simulink model "Roll_OpenLoop"  (R2016b)
settings: Solver=ode3  StartTime=0.0  StopTime=10  FixedStep=.02  RelTol=1e-3  EnableMultiTasking=on
InitFcn:
  | close all
  | clear
  | clc
  | Parameter_Modeling
  | ST=0.02;
  | angle_scale=.0109863;  % 1/91.0222
  | time_scale=.01;
undefined symbols (not defined in the file or in its folder): rad, s
libraries: arduinolib x6, aerolibconvert2 x4, simulink x1
settings Model: SimulationMode=external  ExtModeTrigDuration=2  Creator=Alireza  LastModifiedBy=Ali
settings DataIOCC: LimitDataPoints=on  SaveFormat=Array
settings OptimizationCC: ExpressionDepthLimit=2147483647  MaxStackSize=64
settings DebuggingCC: UnderspecifiedInitializationDetection=Classic  MergeDetectMultiDrivingBlocksExec=none  ParameterTunabilityLossMsg=error  StateNameClashWarn=warning  SFUnexpectedBacktrackingDiag=warning  SFNoUnconditionalDefaultTransitionDiag=warning  SFExecutionAtInitializationDiag=none
settings HardwareCC: ProdBitPerInt=16  ProdBitPerPointer=16  ProdBitPerSizeT=16  ProdBitPerPtrDiffT=16  ProdLargestAtomicFloat=None  ProdWordSize=8  ProdHWDeviceType=Atmel->AVR
settings ModelReferenceCC: PropagateSignalLabelsOutOfModel=off
settings RTWCC: SystemTargetFile=ert.tlc  HardwareBoard=Arduino Mega 2560  TLCOptions=-aInlineSetEventsForThisBaseRateFcn=TLC_FALSE -aRateBasedStepFcn=1 -aSuppressMultiTaskScheduler=TLC_FALSE  TemplateMakefile=ert_default_tmf  Description=Embedded Coder  GenerateReport=on  RTWVerbose=off  Toolchain=Arduino AVR  BuildConfiguration=Faster Runs  IncludeHyperlinkInReport=on  LaunchReport=on  GenerateTraceInfo=on  GenerateTraceReport=on  GenerateTraceReportSl=on  GenerateTraceReportSf=on  GenerateTraceReportEml=on
settings CodeAppCC: ForceParamTrailComments=on  IgnoreCustomStorageClasses=off  OperatorAnnotations=on  SimulinkDataObjDesc=on  SFDataObjDesc=on  MATLABFcnDesc=on  CustomSymbolStrType=$N$R$M  InsertBlockDesc=on  MATLABSourceComments=on  InternalIdentifier=Classic
settings ERTTargetCC: SupportContinuousTime=on  SupportVariableSizeSignals=on
settings ConfigComp: CovMetricSettings=dw  CovHtmlReporting=on  CovSaveCumulativeToWorkspaceVar=on  CovSaveSingleToWorkspaceVar=on  CovExternalEMLEnable=off  CovSFcnEnable=off

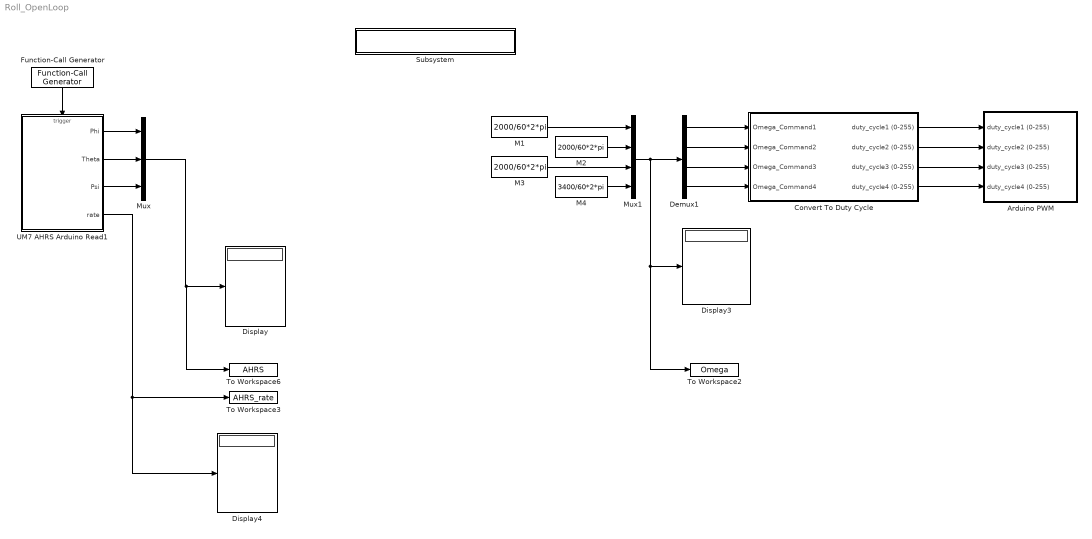
== system Roll_OpenLoop ==
  Arduino PWM : Subsystem  mask{Motor1=8, Motor2=9, Motor3=10, Motor4=11}
      mask prompts: Motor1 "Motor 1 Pin Number"; Motor2 "Motor 2 Pin Number"; Motor3 "Motor 3 Pin Number"; Motor4 "Motor 4 Pin Number"
  Convert To Duty Cycle : Subsystem
  Demux1 : Demux
  Display : Display
  Display3 : Display
  Display4 : Display
  Function-Call Generator : simulink/Ports & Subsystems/Function-Call Generator  sample_time=.02  numberOfIterations=27
  M1 : Constant  Value=2000/60*2*pi
  M2 : Constant  Value=2000/60*2*pi
  M3 : Constant  Value=2000/60*2*pi
  M4 : Constant  Value=3400/60*2*pi
  Mux : Mux  Inputs=3
  Mux1 : Mux
  Subsystem : Subsystem
      settings: OpenFcn=open('Parameter_Modeling')
      mask Display: disp('Edit of the Modeling Parameters')
  To Workspace2 : ToWorkspace  VariableName=Omega  SampleTime=-1
  To Workspace3 : ToWorkspace  VariableName=AHRS_rate  SampleTime=-1
  To Workspace6 : ToWorkspace  VariableName=AHRS  SampleTime=-1
  UM7 AHRS Arduino Read1 : Subsystem  TreatAsAtomicUnit=on
  wires:
  Convert To Duty Cycle/3(duty_cycle3 (0-255)) -> Arduino PWM/3(duty_cycle3 (0-255))
  Convert To Duty Cycle/1(duty_cycle1 (0-255)) -> Arduino PWM/1(duty_cycle1 (0-255))
  Convert To Duty Cycle/4(duty_cycle4 (0-255)) -> Arduino PWM/4(duty_cycle4 (0-255))
  Convert To Duty Cycle/2(duty_cycle2 (0-255)) -> Arduino PWM/2(duty_cycle2 (0-255))
  Function-Call Generator/1 -> UM7 AHRS Arduino Read1/Trigger
  UM7 AHRS Arduino Read1/3(Psi) -> Mux/3
  UM7 AHRS Arduino Read1/2(Theta) -> Mux/2
  UM7 AHRS Arduino Read1/1(Phi) -> Mux/1
  Mux/1 -> To Workspace6/1, Display/1
  Mux1/1 -> To Workspace2/1, Display3/1, Demux1/1
  Demux1/4 -> Convert To Duty Cycle/4(Omega_Command4)
  Demux1/2 -> Convert To Duty Cycle/2(Omega_Command2)
  Demux1/3 -> Convert To Duty Cycle/3(Omega_Command3)
  Demux1/1 -> Convert To Duty Cycle/1(Omega_Command1)
  UM7 AHRS Arduino Read1/4("rate ") -> Display4/1, To Workspace3/1
  M1/1 -> Mux1/1
  M3/1 -> Mux1/3
  M2/1 -> Mux1/2
  M4/1 -> Mux1/4

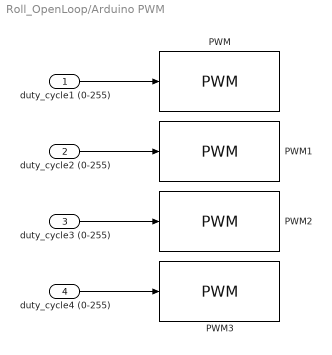
== system Roll_OpenLoop/Arduino PWM ==
  duty_cycle1 (0-255) : Inport
  duty_cycle2 (0-255) : Inport  Port=2
  duty_cycle3 (0-255) : Inport  Port=3
  duty_cycle4 (0-255) : Inport  Port=4
  PWM : arduinolib/PWM  pinNumber=Motor1  blockPlatform=arduino
  PWM1 : arduinolib/PWM  pinNumber=Motor2  blockPlatform=arduino
  PWM2 : arduinolib/PWM  pinNumber=Motor3  blockPlatform=arduino
  PWM3 : arduinolib/PWM  pinNumber=Motor4  blockPlatform=arduino
  wires:
  duty_cycle1 (0-255)/1 -> PWM/1
  duty_cycle2 (0-255)/1 -> PWM1/1
  duty_cycle3 (0-255)/1 -> PWM2/1
  duty_cycle4 (0-255)/1 -> PWM3/1

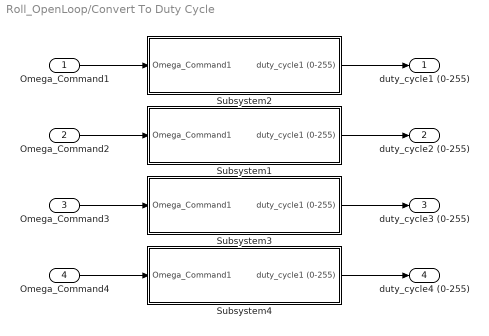
== system Roll_OpenLoop/Convert To Duty Cycle ==
  Omega_Command1 : Inport
  Omega_Command2 : Inport  Port=2
  Omega_Command3 : Inport  Port=3
  Omega_Command4 : Inport  Port=4
  Subsystem1 : Subsystem
  Subsystem2 : Subsystem
  Subsystem3 : Subsystem
  Subsystem4 : Subsystem
  duty_cycle1 (0-255) : Outport
  duty_cycle2 (0-255) : Outport  Port=2
  duty_cycle3 (0-255) : Outport  Port=3
  duty_cycle4 (0-255) : Outport  Port=4
  wires:
  Subsystem1/1(duty_cycle1 (0-255)) -> duty_cycle2 (0-255)/1
  Subsystem3/1(duty_cycle1 (0-255)) -> duty_cycle3 (0-255)/1
  Subsystem4/1(duty_cycle1 (0-255)) -> duty_cycle4 (0-255)/1
  Subsystem2/1(duty_cycle1 (0-255)) -> duty_cycle1 (0-255)/1
  Omega_Command1/1 -> Subsystem2/1(Omega_Command1)
  Omega_Command4/1 -> Subsystem4/1(Omega_Command1)
  Omega_Command3/1 -> Subsystem3/1(Omega_Command1)
  Omega_Command2/1 -> Subsystem1/1(Omega_Command1)

== system Roll_OpenLoop/Subsystem ==

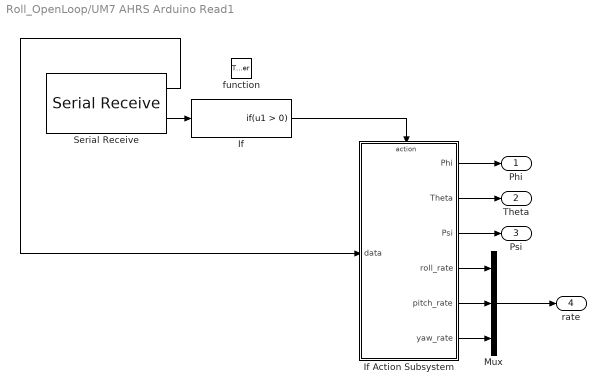
== system Roll_OpenLoop/UM7 AHRS Arduino Read1 ==
  function : TriggerPort  TriggerType=function-call  VariantControl=Variant
  If : If  ShowElse=off
  If Action Subsystem : Subsystem  TreatAsAtomicUnit=on
  Mux : Mux  Inputs=3
  Serial Receive : arduinolib/Serial Receive  portNumber=1  showOutStatus=on  sampleTime=-1  blockPlatform=arduino
  Phi : Outport
  Theta : Outport  Port=2
  Psi : Outport  Port=3
  "rate " : Outport  Port=4
  wires:
  Serial Receive/2 -> If/1
  If/1 -> If Action Subsystem/Action
  Serial Receive/1 -> If Action Subsystem/1(data)
  If Action Subsystem/3(Psi) -> Psi/1
  If Action Subsystem/2(Theta) -> Theta/1
  If Action Subsystem/1(Phi) -> Phi/1
  If Action Subsystem/6(yaw_rate) -> Mux/3
  If Action Subsystem/4(roll_rate) -> Mux/1
  If Action Subsystem/5(pitch_rate) -> Mux/2
  Mux/1 -> "rate "/1

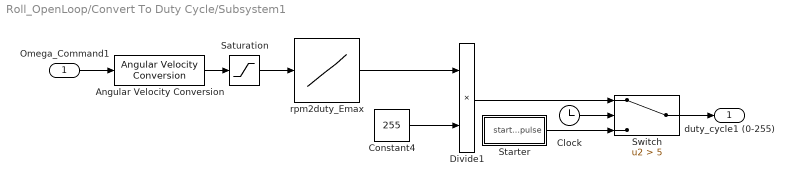
== system Roll_OpenLoop/Convert To Duty Cycle/Subsystem1 ==
  Omega_Command1 : Inport
  Angular Velocity Conversion : aerolibconvert2/Angular Velocity Conversion  IU=rad/s  OU=rpm
  Clock : Clock
  Constant4 : Constant  Value=255
  Divide1 : Product  Inputs=**
  Saturation : Saturate  UpperLimit=6000  LowerLimit=1300
  Starter : Subsystem
  Switch : Switch  Criteria=u2 > Threshold  Threshold=5
  rpm2duty_Emax : Lookup_n-D  NumberOfTableDimensions=1  BreakpointsForDimension1=|  Table=|  RndMeth=Simplest  InputSameDT=on
      BreakpointsForDimension1=|
      | [1201
      | 2305
      | 3096
      | 3930
      | 4118
      | 4555
      | 5122
      | 5552
      | 5957
      | 6291
      | 6360]
      Table=|
      | [0.5
      | 0.55
      | 0.6
      | 0.65
      | 0.7
      | 0.75
      | 0.8
      | 0.85
      | 0.9
      | 0.95
      | 1]
  duty_cycle1 (0-255) : Outport
  wires:
  Divide1/1 -> Switch/1
  Switch/1 -> duty_cycle1 (0-255)/1
  Clock/1 -> Switch/2
  Starter/1(start_pulse) -> Switch/3
  Angular Velocity Conversion/1 -> Saturation/1
  Constant4/1 -> Divide1/2
  Omega_Command1/1 -> Angular Velocity Conversion/1
  rpm2duty_Emax/1 -> Divide1/1
  Saturation/1 -> rpm2duty_Emax/1

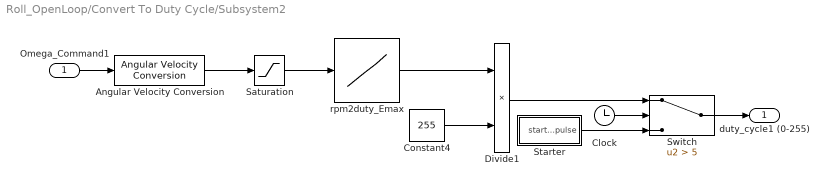
== system Roll_OpenLoop/Convert To Duty Cycle/Subsystem2 ==
  Omega_Command1 : Inport
  Angular Velocity Conversion : aerolibconvert2/Angular Velocity Conversion  IU=rad/s  OU=rpm
  Clock : Clock
  Constant4 : Constant  Value=255
  Divide1 : Product  Inputs=**
  Saturation : Saturate  UpperLimit=6000  LowerLimit=1300
  Starter : Subsystem
  Switch : Switch  Criteria=u2 > Threshold  Threshold=5
  rpm2duty_Emax : Lookup_n-D  NumberOfTableDimensions=1  BreakpointsForDimension1=|  Table=|  RndMeth=Simplest  InputSameDT=on
      BreakpointsForDimension1=|
      | [1201
      | 2305
      | 3096
      | 3930
      | 4118
      | 4555
      | 5122
      | 5552
      | 5957
      | 6291
      | 6360]
      Table=|
      | [0.5
      | 0.55
      | 0.6
      | 0.65
      | 0.7
      | 0.75
      | 0.8
      | 0.85
      | 0.9
      | 0.95
      | 1]
  duty_cycle1 (0-255) : Outport
  wires:
  Omega_Command1/1 -> Angular Velocity Conversion/1
  Constant4/1 -> Divide1/2
  Angular Velocity Conversion/1 -> Saturation/1
  Starter/1(start_pulse) -> Switch/3
  Clock/1 -> Switch/2
  Switch/1 -> duty_cycle1 (0-255)/1
  Divide1/1 -> Switch/1
  rpm2duty_Emax/1 -> Divide1/1
  Saturation/1 -> rpm2duty_Emax/1

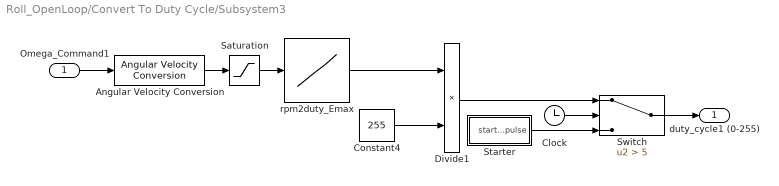
== system Roll_OpenLoop/Convert To Duty Cycle/Subsystem3 ==
  Omega_Command1 : Inport
  Angular Velocity Conversion : aerolibconvert2/Angular Velocity Conversion  IU=rad/s  OU=rpm
  Clock : Clock
  Constant4 : Constant  Value=255
  Divide1 : Product  Inputs=**
  Saturation : Saturate  UpperLimit=6000  LowerLimit=1300
  Starter : Subsystem
  Switch : Switch  Criteria=u2 > Threshold  Threshold=5
  rpm2duty_Emax : Lookup_n-D  NumberOfTableDimensions=1  BreakpointsForDimension1=|  Table=|  RndMeth=Simplest  InputSameDT=on
      BreakpointsForDimension1=|
      | [1201
      | 2305
      | 3096
      | 3930
      | 4118
      | 4555
      | 5122
      | 5552
      | 5957
      | 6291
      | 6360]
      Table=|
      | [0.5
      | 0.55
      | 0.6
      | 0.65
      | 0.7
      | 0.75
      | 0.8
      | 0.85
      | 0.9
      | 0.95
      | 1]
  duty_cycle1 (0-255) : Outport
  wires:
  Omega_Command1/1 -> Angular Velocity Conversion/1
  Constant4/1 -> Divide1/2
  Angular Velocity Conversion/1 -> Saturation/1
  Starter/1(start_pulse) -> Switch/3
  Clock/1 -> Switch/2
  Switch/1 -> duty_cycle1 (0-255)/1
  Divide1/1 -> Switch/1
  rpm2duty_Emax/1 -> Divide1/1
  Saturation/1 -> rpm2duty_Emax/1

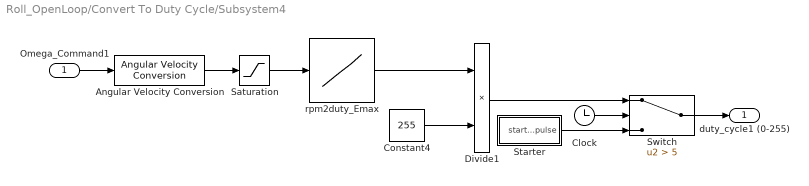
== system Roll_OpenLoop/Convert To Duty Cycle/Subsystem4 ==
  Omega_Command1 : Inport
  Angular Velocity Conversion : aerolibconvert2/Angular Velocity Conversion  IU=rad/s  OU=rpm
  Clock : Clock
  Constant4 : Constant  Value=255
  Divide1 : Product  Inputs=**
  Saturation : Saturate  UpperLimit=6000  LowerLimit=1300
  Starter : Subsystem
  Switch : Switch  Criteria=u2 > Threshold  Threshold=5
  rpm2duty_Emax : Lookup_n-D  NumberOfTableDimensions=1  BreakpointsForDimension1=|  Table=|  RndMeth=Simplest  InputSameDT=on
      BreakpointsForDimension1=|
      | [1201
      | 2305
      | 3096
      | 3930
      | 4118
      | 4555
      | 5122
      | 5552
      | 5957
      | 6291
      | 6360]
      Table=|
      | [0.5
      | 0.55
      | 0.6
      | 0.65
      | 0.7
      | 0.75
      | 0.8
      | 0.85
      | 0.9
      | 0.95
      | 1]
  duty_cycle1 (0-255) : Outport
  wires:
  Divide1/1 -> Switch/1
  Switch/1 -> duty_cycle1 (0-255)/1
  Clock/1 -> Switch/2
  Starter/1(start_pulse) -> Switch/3
  Angular Velocity Conversion/1 -> Saturation/1
  Constant4/1 -> Divide1/2
  Omega_Command1/1 -> Angular Velocity Conversion/1
  rpm2duty_Emax/1 -> Divide1/1
  Saturation/1 -> rpm2duty_Emax/1

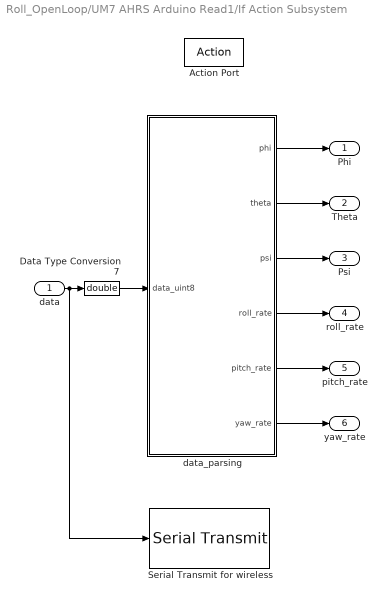
== system Roll_OpenLoop/UM7 AHRS Arduino Read1/If Action Subsystem ==
  data : Inport
  Action Port : ActionPort  ActionType=then
  Data Type Conversion7 : DataTypeConversion  OutDataTypeStr=double
  Serial Transmit for wireless : arduinolib/Serial Transmit  portNumber=2  blockPlatform=arduino
  data_parsing : MATLAB Function  TreatAsAtomicUnit=on
  Phi : Outport
  Theta : Outport  Port=2
  Psi : Outport  Port=3
  roll_rate : Outport  Port=4
  pitch_rate : Outport  Port=5
  yaw_rate : Outport  Port=6
  wires:
  data/1 -> Serial Transmit for wireless/1, Data Type Conversion7/1
  Data Type Conversion7/1 -> data_parsing/1(data_uint8)
  data_parsing/1(phi) -> Phi/1
  data_parsing/2(theta) -> Theta/1
  data_parsing/3(psi) -> Psi/1
  data_parsing/4(roll_rate) -> roll_rate/1
  data_parsing/5(pitch_rate) -> pitch_rate/1
  data_parsing/6(yaw_rate) -> yaw_rate/1

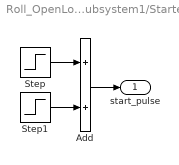
== system Roll_OpenLoop/Convert To Duty Cycle/Subsystem1/Starter ==
  Add : Sum
  Step : Step  After=140
  Step1 : Step  Time=2  After=-30
  start_pulse : Outport
  wires:
  Add/1 -> start_pulse/1
  Step/1 -> Add/1
  Step1/1 -> Add/2

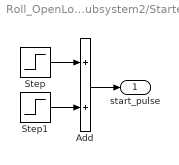
== system Roll_OpenLoop/Convert To Duty Cycle/Subsystem2/Starter ==
  Add : Sum
  Step : Step  After=140
  Step1 : Step  Time=2  After=-30
  start_pulse : Outport
  wires:
  Add/1 -> start_pulse/1
  Step/1 -> Add/1
  Step1/1 -> Add/2

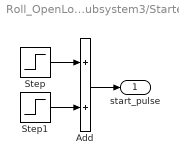
== system Roll_OpenLoop/Convert To Duty Cycle/Subsystem3/Starter ==
  Add : Sum
  Step : Step  After=140
  Step1 : Step  Time=2  After=-30
  start_pulse : Outport
  wires:
  Add/1 -> start_pulse/1
  Step/1 -> Add/1
  Step1/1 -> Add/2

== system Roll_OpenLoop/Convert To Duty Cycle/Subsystem4/Starter ==
  Add : Sum
  Step : Step  After=140
  Step1 : Step  Time=2  After=-30
  start_pulse : Outport
  wires:
  Add/1 -> start_pulse/1
  Step/1 -> Add/1
  Step1/1 -> Add/2

== matlab function Roll_OpenLoop/UM7 AHRS Arduino Read1/If Action Subsystem/data_parsing ==
  data: phi output size=1; data_uint8 input size=1; theta output size=1; psi output size=1; roll_rate output size=1; pitch_rate output size=1; yaw_rate output size=1
function [phi,theta,psi,roll_rate,pitch_rate,yaw_rate] = fcn(data_uint8)
persistent stepp check_sum...
    phi_p theta_p psi_p roll_rate_p pitch_rate_p yaw_rate_p...
    phi_last theta_last psi_last roll_rate_last pitch_rate_last yaw_rate_last;
%% Initialize
if isempty(stepp)
    stepp=0;
    check_sum=0;
    phi_p=0;
    theta_p=0;
    psi_p=0;
    roll_rate_p=0;
    pitch_rate_p=0;
    yaw_rate_p=0;
    phi_last=0;
    theta_last=0;
    psi_last=0;
    roll_rate_last=0;
    pitch_rate_last=0;
    yaw_rate_last=0;
end
angle_scale=.0109863;  % 1/91.0222
rate_scale=1/16;
%% Check Each Byte
if (data_uint8==115 && stepp==0)
    stepp=1;
    check_sum=data_uint8;
elseif(stepp==1 && data_uint8==110)
    stepp=stepp+1;
    check_sum=check_sum+data_uint8;
elseif(stepp==2 && data_uint8==112)
    stepp=stepp+1;
    check_sum=check_sum+data_uint8;
elseif(stepp==3 && data_uint8==212)
    stepp=stepp+1;
    check_sum=check_sum+data_uint8;
elseif(stepp==4 && data_uint8==112)
    stepp=stepp+1;
    check_sum=check_sum+data_uint8;
elseif(stepp==5)
    phi_p=data_uint8*256;
    stepp=stepp+1;
    check_sum=check_sum+data_uint8;
elseif(stepp==6)
    phi_p=phi_p+data_uint8;
    stepp=stepp+1;
    check_sum=check_sum+data_uint8;
elseif(stepp==7)
    theta_p=data_uint8*256;
    stepp=stepp+1;
    check_sum=check_sum+data_uint8;
elseif(stepp==8)
    theta_p=theta_p+data_uint8;
    stepp=stepp+1;
    check_sum=check_sum+data_uint8;
elseif(stepp==9)
    psi_p=data_uint8*256;
    stepp=stepp+1;
    check_sum=check_sum+data_uint8;
elseif(stepp==10)
    psi_p=psi_p+data_uint8;
    stepp=stepp+1;
    check_sum=check_sum+data_uint8;
elseif(stepp==11 || stepp==12)
    if(data_uint8==0)
        stepp=stepp+1;
    else
        stepp=0;
    end
elseif(stepp==13)
    roll_rate_p=data_uint8*256;
    stepp=stepp+1;
    check_sum=check_sum+data_uint8;
elseif(stepp==14)
    roll_rate_p=roll_rate_p+data_uint8;
    stepp=stepp+1;
    check_sum=check_sum+data_uint8;
elseif(stepp==15)
    pitch_rate_p=data_uint8*256;
    stepp=stepp+1;
    check_sum=check_sum+data_uint8;
elseif(stepp==16)
    pitch_rate_p=pitch_rate_p+data_uint8;
    stepp=stepp+1;
    check_sum=check_sum+data_uint8;
elseif(stepp==17)
    yaw_rate_p=data_uint8*256;
    stepp=stepp+1;
    check_sum=check_sum+data_uint8;
elseif(stepp==18)
    yaw_rate_p=yaw_rate_p+data_uint8;
    stepp=stepp+1;
    check_sum=check_sum+data_uint8;
elseif(stepp==19 || stepp==20)
    if(data_uint8==0)
        stepp=stepp+1;
    else
        stepp=0;
    end
elseif(stepp==21 || stepp==22 || stepp==23 || stepp==24)
    stepp=stepp+1;
    check_sum=check_sum+data_uint8;
elseif(stepp==25)
    if (floor(check_sum/256)==data_uint8)
        stepp=stepp+1;
    else
        stepp=0;
    end
elseif(stepp==26)
    if(mod(check_sum,256)==data_uint8)
        phi_last=double(typecast(uint16(phi_p), 'int16'))*angle_scale;
        if mod(phi_last,360)>180;
            phi_last=mod(phi_last,360)-360;
        else
            phi_last=mod(phi_last,360);
        end
        theta_last=double(typecast(uint16(theta_p), 'int16'))*angle_scale;
        if mod(theta_last,360)>180;
            theta_last=mod(theta_last,360)-360;
        else
            theta_last=mod(theta_last,360);
        end
        psi_last=double(typecast(uint16(psi_p), 'int16'))*angle_scale;
        if mod(psi_last,360)>180;
            psi_last=mod(psi_last,360)-360;
        else
            psi_last=mod(psi_last,360);
        end
        roll_rate_last=double(typecast(uint16(roll_rate_p), 'int16'))*rate_scale;
        if mod(roll_rate_last,360)>180;
            roll_rate_last=mod(roll_rate_last,360)-360;
        else
            roll_rate_last=mod(roll_rate_last,360);
        end
        pitch_rate_last=double(typecast(uint16(pitch_rate_p), 'int16'))*rate_scale;
        if mod(pitch_rate_last,360)>180;
            pitch_rate_last=mod(pitch_rate_last,360)-360;
        else
            pitch_rate_last=mod(pitch_rate_last,360);
        end
        yaw_rate_last=double(typecast(uint16(yaw_rate_p), 'int16'))*rate_scale;
        if mod(yaw_rate_last,360)>180;
            yaw_rate_last=mod(yaw_rate_last,360)-360;
        else
            yaw_rate_last=mod(yaw_rate_last,360);
        end
    end
    stepp=0;
end
%% Assign Last True Data to Output
phi=phi_last;
theta=theta_last;
psi=psi_last;
roll_rate=roll_rate_last;
pitch_rate=pitch_rate_last;
yaw_rate=yaw_rate_last;
